simulink model "Boost_Simplified_Model_to_begin"  (R2021a)
settings: Solver=VariableStepAuto  StartTime=0.0  StopTime=10.0  MaxStep=1e-4  RelTol=1e-9
values from neighbouring files (symbols this model uses):
  C = .07e-3    (= 7e-05)    [tranfer_func_ex4.m]
  D_ss = 0.6    [tranfer_func_ex4.m]
  iL_ss = Vo_ss/(R*(1-D_ss))    (= 5.625)    [tranfer_func_ex4.m]
  L = .3e-3    (= 0.0003)    [tranfer_func_ex4.m]
  Vo_ss = V_in/(1-D_ss)    (= 22.5)    [tranfer_func_ex4.m]
undefined symbols (not defined in the file or in its folder): K_LQ
settings Model: Creator=jkord  LastModifiedBy=nikol
settings DebuggingCC: UnconnectedInputMsg=none  UnconnectedOutputMsg=none  UnconnectedLineMsg=none
settings ModelReferenceCC: EnableRefExpFcnMdlSchedulingChecks=off
settings RTWCC: Description=Generic Real-Time Target  GPUComputeCapability=5.0  DLArmComputeVersion=20.02.1

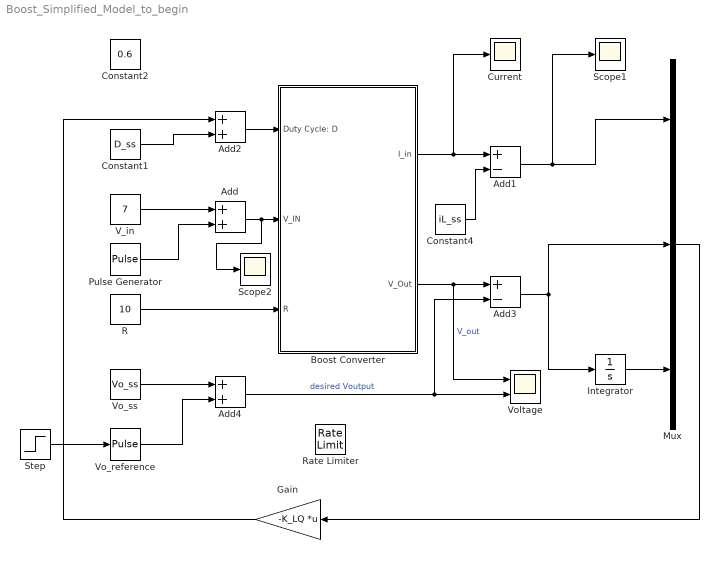
== system Boost_Simplified_Model_to_begin ==
  Add : Sum
  Add1 : Sum  Inputs=+-
  Add2 : Sum
  Add3 : Sum  Inputs=+-
  Add4 : Sum
  Boost Converter : Subsystem
  Constant1 : Constant  Value=D_ss
  Constant2 : Constant  Value=0.6
  Constant4 : Constant  Value=iL_ss
  Current : Scope
  Gain : Gain  Gain=-K_LQ  Multiplication=Matrix(K*u)
  Integrator : Integrator
  Mux : Mux  Inputs=3
  Pulse Generator : DiscretePulseGenerator  PulseType=Time based  Amplitude=5  Period=3  PulseWidth=50  PhaseDelay=1
  R : Constant  Value=10
  Rate Limiter : RateLimiter  RisingSlewLimit=15  FallingSlewLimit=-15  SampleTimeMode=inherited
  Scope1 : Scope
  Scope2 : Scope
  Step : Step  SampleTime=0
  V_in : Constant  Value=7
  Vo_reference : DiscretePulseGenerator  PulseType=Time based  TimeSource=Use external signal  Period=0.5  PulseWidth=50
  Vo_ss : Constant  Value=Vo_ss
  Voltage : Scope  NumInputPorts=2
  wires:
  R/1 -> Boost Converter/3(R)
  Boost Converter/1(I_in) -> Add1/1, Current/1
  Boost Converter/2(V_Out) -> Add3/1, Voltage/1  "V_out"
  Add/1 -> Scope2/1, Boost Converter/2(V_IN)
  V_in/1 -> Add/1
  Pulse Generator/1 -> Add/2
  Add2/1 -> Boost Converter/1(Duty Cycle: D)
  Constant1/1 -> Add2/2
  Gain/1 -> Add2/1
  Vo_ss/1 -> Add4/1
  Vo_reference/1 -> Add4/2
  Add4/1 -> Add3/2, Voltage/2  "desired Voutput"
  Constant4/1 -> Add1/2
  Add3/1 -> Mux/2, Integrator/1
  Integrator/1 -> Mux/3
  Add1/1 -> Scope1/1, Mux/1
  Mux/1 -> Gain/1
  Step/1 -> Vo_reference/1

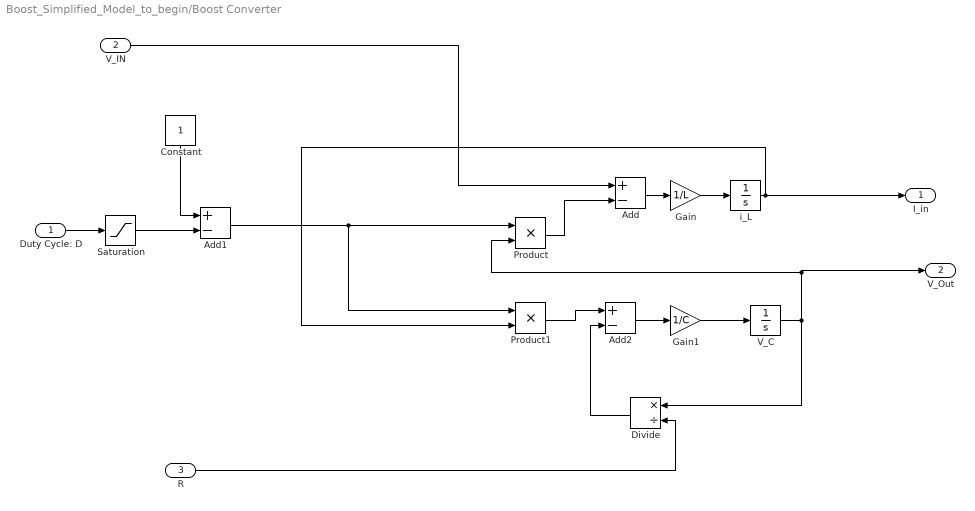
== system Boost_Simplified_Model_to_begin/Boost Converter ==
  Duty Cycle: D : Inport
  V_IN : Inport  Port=2
  R : Inport  Port=3
  Add : Sum  Inputs=+-
  Add1 : Sum  Inputs=+-
  Add2 : Sum  Inputs=+-
  Constant : Constant
  Divide : Product  Inputs=*/
  Gain : Gain  Gain=1/L
  Gain1 : Gain  Gain=1/C
  Product : Product
  Product1 : Product
  Saturation : Saturate  UpperLimit=0.9  LowerLimit=0.1
  V_C : Integrator  InitialCondition=10
  i_L : Integrator  InitialCondition=2
  I_in : Outport
  V_Out : Outport  Port=2
  wires:
  Product/1 -> Add/2
  i_L/1 -> I_in/1, Product1/2
  Gain1/1 -> V_C/1
  V_IN/1 -> Add/1
  Gain/1 -> i_L/1
  V_C/1 -> Divide/1, V_Out/1, Product/2
  Add/1 -> Gain/1
  Product1/1 -> Add2/1
  Add2/1 -> Gain1/1
  Divide/1 -> Add2/2
  R/1 -> Divide/2
  Duty Cycle: D/1 -> Saturation/1
  Saturation/1 -> Add1/2
  Constant/1 -> Add1/1
  Add1/1 -> Product1/1, Product/1
